simulink model "boat_dynamics_model"  (R2025a)
settings: Solver=ode4  StartTime=0.0  StopTime=15  FixedStep=Ts_sim  RelTol=1e-3
values from neighbouring files (symbols this model uses):
  ctrl_params =     [boat_controller_parameters.mat]    (also in setup_MDL.m = boat_controller_parameters())
  plant_params = boat_model_parameters_4dof()    [setup_MDL.m]
  trim =     [last_trim.mat]    (also in setup_RL.m = data.trim; tmp_trim_4dof.mat)
  u0 = u0(:)    [find_A_B_LQR.m]    (also in setup_MDL.m = trim.u0; setup_RL.m = trim.u0; tmp_continuous_controller.mat = [4.86274582601 4.86274582601 5.08309482386 4.40845063905]; tmp_discrete_augumented_LQI_controller.mat = [4.86274582601 4.86274582601 5.08309482386])
  x0 = x0(:)    [find_A_B_LQR.m]    (also in setup_MDL.m = trim.x0; setup_RL.m = trim.x0; tmp_continuous_controller.mat = [0 2.5 -0.1 0 0 0 0 0 0 0 4.86274582601 4.86274582601 ... (1; tmp_discrete_controller.mat = [0 2.5 -0.1 0 0 0 0 0 0 0 4.86274582601 4.86274582601 ... (1)
undefined symbols (not defined in the file or in its folder): Ts_sim
libraries: simulink_extras x4, sim3dlib x2, rllib x1
(part 2 of 2)

== matlab function boat_dynamics_model/LQR discrete augumented ==
  data: xi_ output; reference input; velocity input size=1; x_hat input size=[11 1]; delay_states input size=[12 1]; u output; params input
function [xi_, u] = lq_discrete_augumented_controller(reference, velocity, x_hat, delay_states, params) %#codegen

    % Gain scheduling data
    velocity_grid = params.controller.LQ.velocity_grid;
    K_grid  = params.controller.LQ.K_aug_lqi_grid;
    x0_grid = params.controller.LQ.x0aug_grid;
    u0_grid = params.controller.LQ.u0_grid;
    Nv = numel(velocity_grid);

    % Find scheduling interval
    % Clamp below scheduling range
    if velocity <= velocity_grid(1)
        K  = K_grid(:,:,1);
        x0 = x0_grid(:,1);
        u0 = u0_grid(:,1);
    % Clamp above scheduling range
    elseif velocity >= velocity_grid(Nv)
        K  = K_grid(:,:,Nv);
        x0 = x0_grid(:,Nv);
        u0 = u0_grid(:,Nv);
    else
        % Find V_i <= V < V_{i+1}
        idx = 1;
        for i = 1:Nv-1
            if velocity >= velocity_grid(i) && ...
               velocity <  velocity_grid(i+1)

                idx = i;
                break;
            end
        end
        V1 = velocity_grid(idx);
        V2 = velocity_grid(idx+1);

        % Linear interpolation coefficient
        mu = (velocity - V1) / (V2 - V1);
        % Interpolate controller and trim point
        K = (1 - mu) * K_grid(:,:,idx) + ...
                 mu  * K_grid(:,:,idx+1);
        x0 = (1 - mu) * x0_grid(:,idx) + ...
                  mu  * x0_grid(:,idx+1);
        u0 = (1 - mu) * u0_grid(:,idx) + ...
                  mu  * u0_grid(:,idx+1);
    end

    % Current estimated state
    % x_hat contains yaw states at indices 5 and 8 -> remove them
    %
    % resulting state:
    % [z zdot phi theta p q delta_FL delta_FR delta_R]
    x = x_hat([1 2 3 4 6 7 9 10 11]);
    % Add actuator transport-delay states
    x = [x; delay_states];

    % Apply commanded references
    % reference:
    % [z_ref;
    %  phi_ref;
    %  theta_ref]
    x0(1) = reference(1);   % zW / heave
    x0(3) = reference(2);   % phi / roll
    x0(4) = reference(3);   % theta / pitch

    % Integrate the roll pitch and heave error numerically
    persistent xi
    if isempty(xi)
        xi = zeros(3,1);
    end
    % integrate
    xi = xi + params.Ts * [ ...
        x(1) - reference(1); ... % zW / heave
        x(3) - reference(2); ... % phi / roll
        x(4) - reference(3) ...  % theta / pitch
    ];
    xi_=xi;

    % State error
    dx = x - x0;
    % integral part extension
    dx = [dx; xi];
    % LQ control
    du = -K * dx;
    % Full actuator command
    u = u0 + du;

end
%     % Load once (persistent)
%     persistent K u0 x0 ix iu
%     if isempty(K)
%         data = load('tmp_discrete_augumented_controller.mat');
%         K  = data.Kaug;
%         u0 = data.u0;
%         x0 = data.x0aug;
%     end
% 
%     % x_hat contains yaw states at 5 and 8th idxes filter them out
%     % [z zdot phi theta p q delta_FL delta_FR delta_R]
%     x = x_hat([1 2 3 4   6 7   9 10 11]);
% 
%     % augument x with actuator delay states
%     x = [x; delay_states];
% 
%     % Reference aka setpoint parameters.. could be commented out if not necessary
%     x0(1) = reference(1); % zW aka heave
%     x0(3) = reference(2); % phi aka roll
%     x0(4) = reference(3); % theta aka pitch
% 
%     % State error
%     dx = x - x0;
% 
%     % LQR control
%     du = -K * dx;
% 
%     % Full control input
%     u = u0 + du;
% end

== matlab function boat_dynamics_model/LQR continuous ==
  data: dx output; du output; x input; u output
function [dx, du, u] = lqr_controller(x) %#codegen

    % Load once (persistent)
    persistent K u0 x0 ix iu
    if isempty(K)
        data = load('tmp_continuous_controller.mat');
        % data = load('tmp_discrete_controller.mat');
        K  = data.K;
        u0 = data.u0;
        x0 = data.x0;
        ix = data.ix;
        iu = data.iu;
    end
    
    % State error
    dx = x - x0;
    
    % LQR control  (only selected states)
    du = -K * dx(ix);
    
    % Full control input
    u = u0;
    u(1:3) = u0(1:3) + du;   % only flap commands
end
